simulink model "visual_map_model"  (R2018b)
settings: Solver=VariableStepAuto  StartTime=0.0  StopTime=10000.0  RelTol=1e-3
settings Model: Creator=kchu02  LastModifiedBy=kchu02
settings DataIOCC: ExternalInput=untitled.getElement('roll'),untitled.getElement('pitch'),untitled.getElement('heading')  LoadExternalInput=on

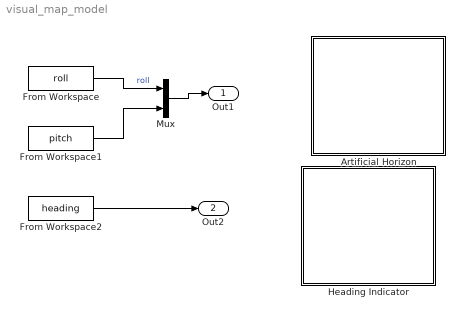
== system visual_map_model ==
  Artificial Horizon : Subsystem  DialogController=aeroblksHMICreateDDGDialog  IsWebBlock=on  mask(MWDashboardBlock){webBlockId=8c9f987b-9b09-44ab-862a-b82b652a9664, webBlockType=artificialhorizon, ShowInLibBrowser=on, ShowInitialText=on, HMISrcModelName=visual_map_model}
      mask prompts: webBlockId "WebBlock Id"; webBlockType "WebBlock Type"; HMISrcModelName "Source Model"
      mask help: aeroblksHMI:aeroblkhmi:ArtificialHorizonDialogDesc
      mask Help: eval('asbhmihelp(''artificialhorizon'')');
      mask Display:
      | if strcmp(get_param(bdroot(gcb),'BlockDiagramType'), 'library')
      |  image([(matlabroot) '/toolbox/aeroblks/aeroblks/hmi/icons/ArtificialHorizonIcon.svg'])
      | end
  From Workspace : FromWorkspace  VariableName=roll  OutDataTypeStr=double  SampleTime=0
  From Workspace1 : FromWorkspace  VariableName=pitch  OutDataTypeStr=double  SampleTime=0
  From Workspace2 : FromWorkspace  VariableName=heading  OutDataTypeStr=double  SampleTime=0
  Heading Indicator : Subsystem  DialogController=aeroblksHMICreateDDGDialog  IsWebBlock=on  mask(MWDashboardBlock){webBlockId=1a92d5a3-7f54-4e7e-8610-30ca7e9d3303, webBlockType=headingindicator, ShowInLibBrowser=on, ShowInitialText=on, HMISrcModelName=visual_map_model}
      mask prompts: webBlockId "WebBlock Id"; webBlockType "WebBlock Type"; HMISrcModelName "Source Model"
      mask help: aeroblksHMI:aeroblkhmi:HeadingIndicatorDialogDesc
      mask Help: eval('asbhmihelp(''headingindicator'')');
      mask Display:
      | if strcmp(get_param(bdroot(gcb),'BlockDiagramType'), 'library')
      |  image([(matlabroot) '/toolbox/aeroblks/aeroblks/hmi/icons/HeadingIndicatorIcon.svg'])
      | end
  Mux : Mux  Inputs=2
  Out1 : Outport
  Out2 : Outport  Port=2
  wires:
  From Workspace/1 -> Mux/1  "roll"
  Mux/1 -> Out1/1
  From Workspace1/1 -> Mux/2
  From Workspace2/1 -> Out2/1

== system visual_map_model/Artificial Horizon ==

== system visual_map_model/Heading Indicator ==
